simulink model "Eval_Test_values"  (Simulink 7.5)
settings: Solver=VariableStepDiscrete  StartTime=0.0  StopTime=5.5  RelTol=1e-3
undefined symbols (not defined in the file or in its folder): sigbuilder_block
settings Model: Creator=Robert  LastModifiedBy=Anonymos  BufferReuse=off
settings OptimizationCC: OptimizeBlockIOStorage=off  BufferReuse=off  ExpressionFolding=off  LocalBlockOutputs=off  InitFltsAndDblsToZero=on
settings DebuggingCC: SaveWithParameterizedLinksMsg=none  SignalResolutionControl=TryResolveAllWithWarning  MultiTaskDSMMsg=warning  MultiTaskCondExecSysMsg=none  StrictBusMsg=Warning
settings RTWCC: IncludeERTFirstTime=on
settings GRTTargetCC: TargetFcnLib=ansi_tfl_tmw.mat

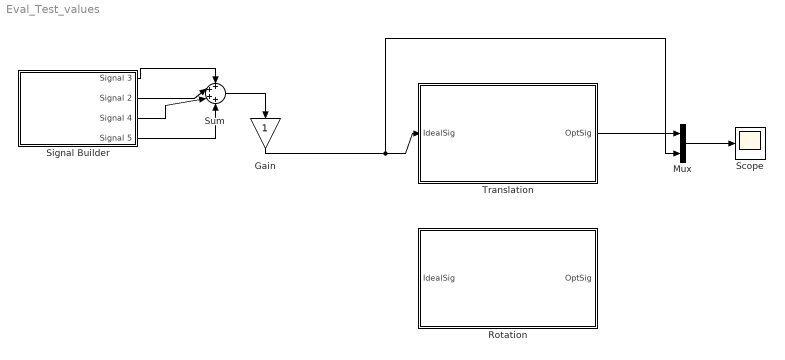
== system Eval_Test_values ==
  Gain : Gain  ParameterDataType=fixdt(1, 16)  ParameterScaling=2^0  OutDataType=fixdt(1, 16)  OutScaling=2^0
  Mux : Mux  Inputs=2
  Rotation : Subsystem  mask{Opt_Var=0.000134, Opt_Var_ST=0.001, Opt_Limit=5, Opt_Delay=0.1, Opt_ST=0.1, Opt_Ori_SG=0.2}
      mask prompts: Opt_Var "Variance"; Opt_Var_ST "Sample Time of Variance"; Opt_Limit "Limitation [m/s]"; Opt_Delay "Delay"; Opt_ST "Sample Time (1/Frame Rate)"; Opt_Ori_SG "Original Signal Gain"
  Scope : Scope
      settings: TickLabels=off  YMin=0  YMax=0.2  SampleInput=on
  Signal Builder : Subsystem  Tag=STV Subsys  LoadFcn=sigbuilder_block('load');  StartFcn=sigbuilder_block('start');  StopFcn=sigbuilder_block('stop');  ClipboardFcn=sigbuilder_block('clipboard');  mask(Sigbuilder block){}
      mask help: Create and generate interchangeable groups of signals whose waveforms are piecewise linear.
      mask init:
      | if ~strcmp(get_param(bdroot(gcbh),'SimulationStatus'),'stopped') tuvar = sigbuilder_block('maskInit'); end
      settings: CopyFcn=sigbuilder_block('copy');  DeleteFcn=sigbuilder_block('delete');  ModelCloseFcn=sigbuilder_block('modelClose');  PreSaveFcn=sigbuilder_block('preSave');  NameChangeFcn=sigbuilder_block('namechange');  OpenFcn=sigbuilder_block('open',[437.25 199.5 550.5 399.75 ]);  CloseFcn=sigbuilder_block('close');
      mask Display: plot(0,0,100,100,[10,10,40,40,10],[80,20,20,80,80],[40,10],[50,50], [40,27,10],[65,72,56],[40,25,25,10],[28,28,43,43]);
  Sum : Sum  Inputs=++++  OutDataType=fixdt(1, 16)  OutScaling=2^0
  Translation : Subsystem  mask{Opt_Var=0.000134, Opt_Var_ST=0.001, Opt_Limit=5, Opt_Delay=0.1, Opt_ST=0.1, Opt_Ori_SG=0.2}
      mask prompts: Opt_Var "Variance"; Opt_Var_ST "Sample Time of Variance"; Opt_Limit "Limitation [m/s]"; Opt_Delay "Delay"; Opt_ST "Sample Time (1/Frame Rate)"; Opt_Ori_SG "Original Signal Gain"
  wires:
  Signal Builder/1(Signal 3) -> Sum/1
  Signal Builder/2(Signal 2) -> Sum/2
  Signal Builder/3(Signal 4) -> Sum/3
  Signal Builder/4(Signal 5) -> Sum/4
  Sum/1 -> Gain/1
  Mux/1 -> Scope/1
  Gain/1 -> Translation/1(IdealSig), Mux/2
  Translation/1(OptSig) -> Mux/1

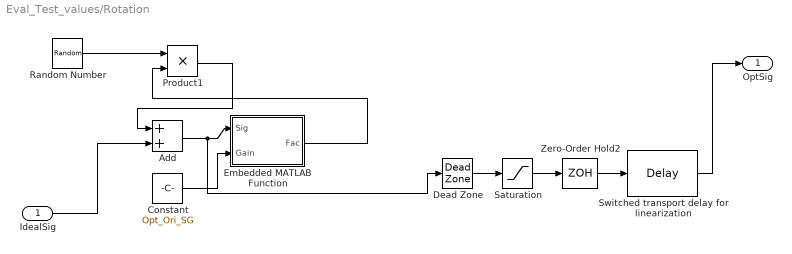
== system Eval_Test_values/Rotation ==
  IdealSig : Inport  OutDataType=fixdt(1, 16)  OutScaling=2^0
  Add : Sum  OutDataType=fixdt(1, 16)  OutScaling=2^-10
  Constant : Constant  Value=Opt_Ori_SG  OutDataType=fixdt(1, 16)  OutScaling=2^0
  Dead Zone : DeadZone  LowerValue=0  UpperValue=0  SaturateOnIntegerOverflow=on
  Embedded MATLAB Function : Stateflow chart  TreatAsAtomicUnit=on
  Product1 : Product  OutDataType=fixdt(1, 16)  OutScaling=2^0  RndMeth=Zero
  Random Number : RandomNumber  Variance=Opt_Var  Seed=234234  SampleTime=Opt_Var_ST
  Saturation : Saturate  UpperLimit=Opt_Limit  LowerLimit=-Opt_Limit  OutDataType=fixdt(1, 16)  OutScaling=2^0
  Switched transport delay for linearization : TransportDelay  DelayTime=Opt_Delay  PadeOrder=2
  Zero-Order Hold2 : ZeroOrderHold  SampleTime=Opt_ST
  OptSig : Outport  OutDataType=fixdt(1, 16)  OutScaling=2^0
  wires:
  Add/1 -> Embedded MATLAB Function/1(Sig), Dead Zone/1
  Embedded MATLAB Function/1(Fac) -> Product1/2
  Product1/1 -> Add/1
  Saturation/1 -> Zero-Order Hold2/1
  Dead Zone/1 -> Saturation/1
  Zero-Order Hold2/1 -> Switched transport delay for linearization/1
  Random Number/1 -> Product1/1
  Switched transport delay for linearization/1 -> OptSig/1
  IdealSig/1 -> Add/2
  Constant/1 -> Embedded MATLAB Function/2(Gain)

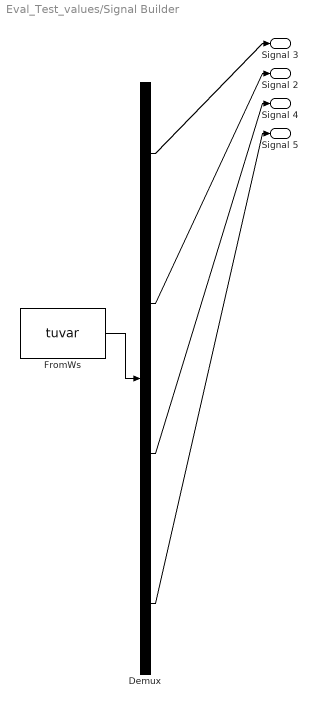
== system Eval_Test_values/Signal Builder ==
  Demux : Demux  Tag=STV Demux
  FromWs : FromWorkspace  Tag=STV FromWs  VariableName=tuvar  SampleTime=0  SigBuilderData=DataTag0  VnvData=DataTag1
      SigBuilderData=|
      | common.afterFinalStr = 'Extrapolate'
      | common.sampleTime = 0
      | dataSet.timeRange = [0 7]
      | dataSet.name = 'Group 1'
      | sbobj.Groups.Name = 'Group 1'
      | sbobj.Groups.Signals(1).Name = 'Signal 3'
      | sbobj.Groups.Signals(1).XData = [0 0.1 0.1 0.6 0.6 7]
      | sbobj.Groups.Signals(1).YData = [0 0 0.1 0.1 0 0]
      | sbobj.Groups.Signals(2).Name = 'Signal 2'
      | sbobj.Groups.Signals(2).XData = [0 0.8 0.8 1.3 1.3 7]
      | sbobj.Groups.Signals(2).YData = [0 0 0.2 0.2 0 0]
      | sbobj.Groups.Signals(3).Name = 'Signal 4'
      | sbobj.Groups.Signals(3).XData = [0 1.5 3.5 3.5 7]
      | sbobj.Groups.Signals(3).YData = [0 0 0.2 0 0]
      | sbobj.Groups.Signals(4).Name = 'Signal 5'
      | sbobj.Groups.Signals(4).XData = [0 1 2 3 4 4.1 4.2 4.3 4.4 4.5 4.6 4.7 4.86 4.86 7]
      | sbobj.Groups.Signals(4).YData = [0 0 0 0 0 0 0.005 0.01 0.02 0.03 0.045 0.09 0.2 0 0]
  Signal 3 : Outport  Tag=STV Outport
  Signal 2 : Outport  Tag=STV Outport  Port=2
  Signal 4 : Outport  Tag=STV Outport  Port=3
  Signal 5 : Outport  Tag=STV Outport  Port=4
  wires:
  FromWs/1 -> Demux/1
  Demux/1 -> Signal 3/1
  Demux/2 -> Signal 2/1
  Demux/3 -> Signal 4/1
  Demux/4 -> Signal 5/1

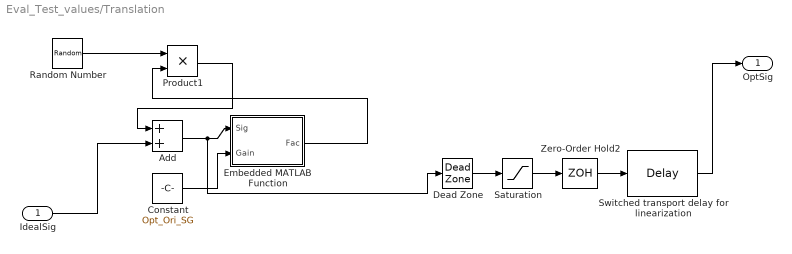
== system Eval_Test_values/Translation ==
  IdealSig : Inport  OutDataType=fixdt(1, 16)  OutScaling=2^0
  Add : Sum  OutDataType=fixdt(1, 16)  OutScaling=2^-10
  Constant : Constant  Value=Opt_Ori_SG  OutDataType=fixdt(1, 16)  OutScaling=2^0
  Dead Zone : DeadZone  LowerValue=0  UpperValue=0  SaturateOnIntegerOverflow=on
  Embedded MATLAB Function : Stateflow chart  TreatAsAtomicUnit=on
  Product1 : Product  OutDataType=fixdt(1, 16)  OutScaling=2^0  RndMeth=Zero
  Random Number : RandomNumber  Variance=Opt_Var  Seed=234234  SampleTime=Opt_Var_ST
  Saturation : Saturate  UpperLimit=Opt_Limit  LowerLimit=-Opt_Limit  OutDataType=fixdt(1, 16)  OutScaling=2^0
  Switched transport delay for linearization : TransportDelay  DelayTime=Opt_Delay  PadeOrder=2
  Zero-Order Hold2 : ZeroOrderHold  SampleTime=Opt_ST
  OptSig : Outport  OutDataType=fixdt(1, 16)  OutScaling=2^0
  wires:
  Add/1 -> Embedded MATLAB Function/1(Sig), Dead Zone/1
  Embedded MATLAB Function/1(Fac) -> Product1/2
  Product1/1 -> Add/1
  Saturation/1 -> Zero-Order Hold2/1
  Dead Zone/1 -> Saturation/1
  Zero-Order Hold2/1 -> Switched transport delay for linearization/1
  Random Number/1 -> Product1/1
  Switched transport delay for linearization/1 -> OptSig/1
  IdealSig/1 -> Add/2
  Constant/1 -> Embedded MATLAB Function/2(Gain)

== matlab function Rotation/Embedded MATLAB Function ==
  data: Sig input double; Fac output double; Gain input double
function Fac = fcn(Sig, Gain)
%#eml

Fac=Sig/Gain;

== matlab function Translation/Embedded MATLAB Function ==
  data: Sig input double; Fac output double; Gain input double
function Fac = fcn(Sig, Gain)
%#eml

Fac=Sig/Gain;
